simulink model "Mixer_LUT_Ex1"  (R2023a)
settings: Solver=VariableStepAuto  StartTime=0.0  StopTime=0.2  RelTol=1e-3
undefined symbols (not defined in the file): None, S, vsva2197, xcvc1902
libraries: dspsrcs4 x2, aieDSP x1, dspsigops x1, vmcUtilities x1
settings Model: Creator=sdegala  LastModifiedBy=robg
settings ModelReferenceCC: EnableRefExpFcnMdlSchedulingChecks=on

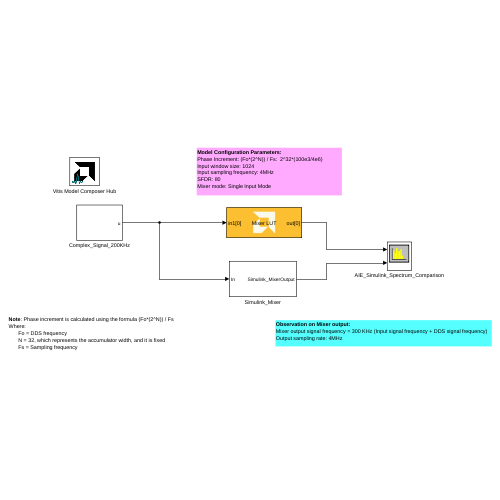
[thumbnail: Simulink's stored preview of the top-level diagram]
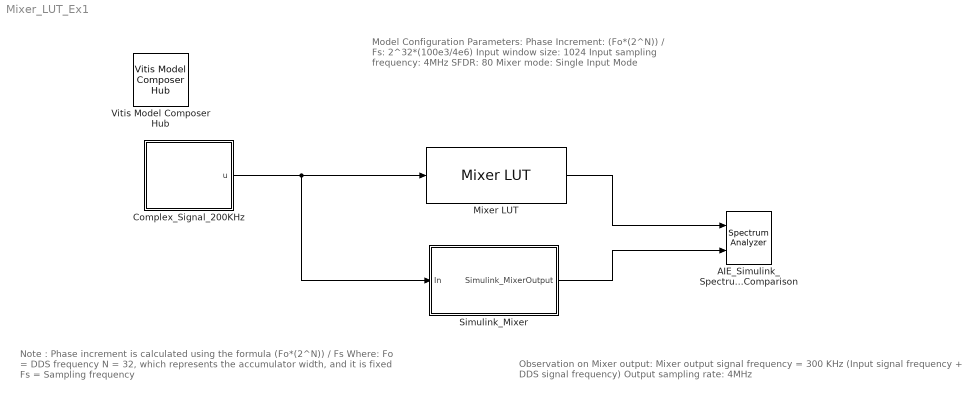
== system Mixer_LUT_Ex1 ==
  note: Observation on Mixer output:
      | Mixer output signal frequency = 300 KHz (Input signal frequency + DDS signal frequency)
      | Output sampling rate: 4MHz
  note: Model Configuration Parameters:
      | Phase Increment: (Fo*(2^N)) / Fs: 2^32*(100e3/4e6)
      | Input window size: 1024
      | Input sampling frequency: 4MHz
      | SFDR: 80
      | Mixer mode: Single Input Mode
  note: Note : Phase increment is calculated using the formula (Fo*(2^N)) / Fs
      | Where:
      | Fo = DDS frequency
      | N = 32, which represents the accumulator width, and it is fixed
      | Fs = Sampling frequency
  AIE_Simulink_Spectrum_Comparison : SpectrumAnalyzer  NumInputPorts=2  AveragingMethod=Exponential  ShowLegend=on  ChannelNames="[\"\"]"  DefaultConfigurationName=spbscopes.SpectrumAnalyzerBlockCfg
  Complex_Signal_200KHz : Subsystem
  Mixer LUT : aieDSP/Mixer LUT  AIE_VARIANT=1  data_type=cfloat  mixer_mode=Single Input Mode  sfdr=80  ssr=1  input_window_size=1024  USE_PHASE_RELOAD=off  phase_increment=1.0737e+08  initial_phase_offset=0  rnd_mode=Floor  sat_mode=0-None  blockJsonConstraints=[]  blockJsonConstraintsInternal=[]  spec=vmc_mixer_lut.json  SerializedMaskParamNames=[]  SerializedMaskParamValues=[]  SerializedMaskParamVisibilities=[]  block_type=Mixer LUT  SerializedMaskParamDataypes=uint|typename|uint|uint|uint|uint|bool|uint|uint|uint|uint  SerializedMaskParamEnumStrArr=0|0|Single Input Mode,Dual Input Mode|0|0|0|0|0|0|Floor,Ceiling,Round to positive infinity,Round to negative infinity,Round symmetrical to infinity,Round symmetrical to zero,Round convergent to even,Round convergent to odd|0-None,1-Asymmetric,3-Symmetric  SerializedMaskParamEnumValArr=0|0|1,2|0|0|0|0|0|0|0,1,2,3,4,5,6,7|0,1,3  SerializedMaskParamVectorArr=0|0|0|0|0|0|0|0|0|0|0
  Simulink_Mixer : Subsystem
  Vitis Model Composer Hub : vmcUtilities/Vitis Model Composer Hub  Tag=genX  CodeGeneration=off  StartColumn=1  NumberOfColumns=1  TargetDirectory=./code  exportDesign=off  analyzeDesign=off  validateDesignOnHw=off  ExportType=AI Engines  IpVendor=xilinx.com  IpLibrary=hls  IpVersion=1.0  IpHWLanguage=Verilog  AieCompilerOptions={}  AieSimulatorOptions={}  CreateTestbench=off  TestbenchStackSize=10  RunRtlSim=off  RunCSim=off  RunAieSim=off  AieSimTimeout=50000  RunAieSimProfiling=off  LaunchVitisAnalyzer=off  PlotOutput=off  RunX86Sim=off  X86SimTimeout=10  GenHwImage=off  GenLibadfXo=off  GenHwValidationCode=off  PlatformType=Not Specified  HwSystemType=Baremetal  HwValidationTarget=hw  ProjDevice=xcvc1902-vsva2197-1LP-e-S  ProjDevicePart=xcvc1902-vsva2197-1LP-e-S  AIEType=AIE  SamplePeriod=-1  ClockFrequency=200  DataPathParallelism=1  xilinxfamily=versalaicore  part=xcvc1902  speed=-1LP-e-S  package=vsva2197  directory=./netlist  testbench=off  incr_netlist=off  synthesis_tool=Vivado  clock_wrapper=Clock Enables  dbl_ovrd=According to Block Masks  dcm_input_clock_period=10  sysclk_period=10  simulink_period=1  eval_field=0  LogFileName=''  NThreads=4
  wires:
  Complex_Signal_200KHz/1(u) -> Simulink_Mixer/1(In), Mixer LUT/1
  Mixer LUT/1 -> AIE_Simulink_Spectrum_Comparison/1
  Simulink_Mixer/1(Simulink_MixerOutput) -> AIE_Simulink_Spectrum_Comparison/2

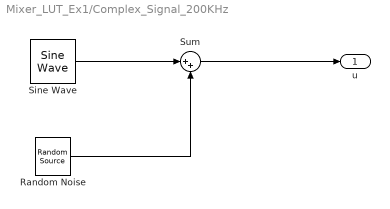
== system Mixer_LUT_Ex1/Complex_Signal_200KHz ==
  Random Noise : dspsrcs4/Random Source  SrcType=Gaussian  NormMethod=Ziggurat  CltLength=12  MinVal=0  MaxVal=1  MeanVal=0  VarVal=1e-3  RepMode=Not repeatable  rawSeed=1  IsInherit=off  SampMode=Discrete  SampTime=1/4e6  SampFrame=1024  DataType=Single  OutComplex=Real  OutputFrames=off
  Sine Wave : dspsrcs4/Sine Wave  Amplitude=1  Frequency=200e3  Phase=0  SampleMode=Discrete  OutComplex=Complex  CompMethod=Trigonometric fcn  TableSize=Speed  SampleTime=1/4e6  SamplesPerFrame=1024  ResetState=Restart at time zero  OutputFrames=off  dataType=single  wordLen=16  udDataType=sfix(16)  fracBitsMode=Best precision  numFracBits=15  OutDataTypeStr=single  LastOutDataTypeStr=single
  Sum : Sum  Inputs=|++
  u : Outport
  wires:
  Sine Wave/1 -> Sum/1
  Sum/1 -> u/1
  Random Noise/1 -> Sum/2

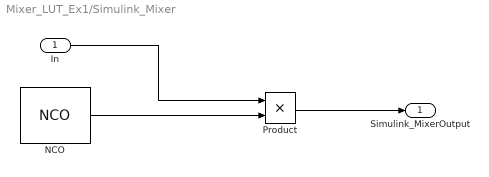
== system Mixer_LUT_Ex1/Simulink_Mixer ==
  In : Inport
  NCO : dspsigops/NCO  AccIncSrc=Specify via dialog  AccInc=1.0737e+08  PhaseOffsetSrc=Specify via dialog  PhaseOffset=0  AccumWL=32  HasDither=off  DitherWL=4  PNgeneratorLength=19  HasPhaseQuantizer=on  TableDepth=16  HasOutputPhaseError=off  Formula=Complex exponential  DataType=single  OutputWL=16  OutputFL=14  CompMethod=Table lookup (no interpolation)  SampleTime=1/4e6  SamplesPerFrame=1024  OutputFrames=off
  Product : Product
  Simulink_MixerOutput : Outport
  wires:
  NCO/1 -> Product/2
  In/1 -> Product/1
  Product/1 -> Simulink_MixerOutput/1
